simulink model "bench_axle"  (R2024b)
settings: Solver=daessc  StartTime=0.0  StopTime=20  MaxStep=1e-3  RelTol=1e-3
values from neighbouring files (symbols this model uses):
  PN = evalin('base','PN')    [run_bench_string_heat.m]
libraries: fl_lib x11, loco_native_lib x10, nesl_utility x8, sdl_lib x1
settings Model: Creator=BillBeverley  LastModifiedBy=BillBeverley

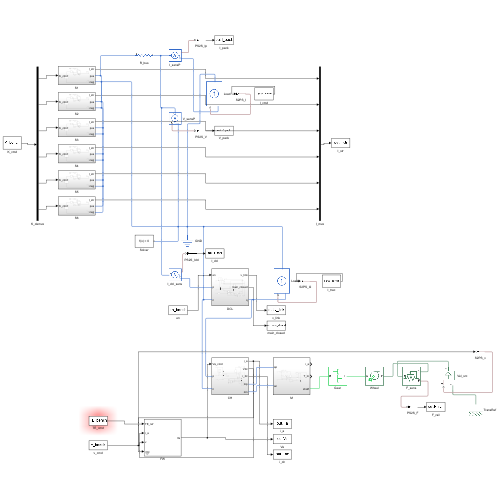
[thumbnail: Simulink's stored preview of the top-level diagram]
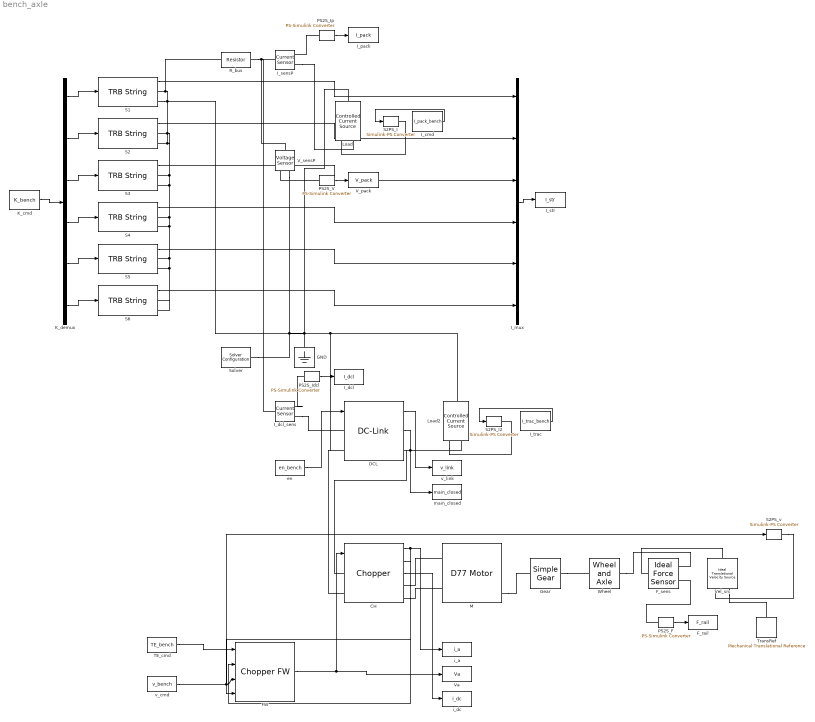
== system bench_axle ==
  CH : loco_native_lib/Chopper  SystemSampleTime=-1  VariantActivationTime=update diagram  AllowFlexibleInterface=on  Latency=0  AutoFrameSizeCalculation=off
  DCL : loco_native_lib/DC-Link  SystemSampleTime=-1  VariantActivationTime=update diagram  AllowFlexibleInterface=on  Latency=0  AutoFrameSizeCalculation=off
  FW : loco_native_lib/Chopper FW  A=PN.ax
  F_rail : ToWorkspace  VariableName=F_rail  SaveFormat=Timeseries  SampleTime=-1
  F_sens : fl_lib/Mechanical/Mechanical Sensors/Ideal Force Sensor
  GND : fl_lib/Electrical/Electrical Elements/Electrical Reference
  Gear : sdl_lib/Gears/Simple Gear  ratio=PN.ax.G  rotation_direction=sdl.enum.shaftOutputDirection.same  friction_model=sdl.enum.gear_efficiencies_load.constant  T_noload=0.1 N*m  T_nom=5 N*m  efficiency_nom=0.8  efficiency=PN.ax.eta_g  temperature_TLU=[280, 300, 320] K  load_TLU=[1, 5, 10] N*m  efficiency_TLU=[.95, .9, .85]  efficiency_TLU2=[.85, .8, .75; .95, .9, .85; .85, .8, .7]  w_thr=0.01 rad/s  pwr_thr=1e3 W  enable_backlash=false  hardstop_model=simscape.enum.hardstop.smooth  backlash_distance=1e-3 mm  r_base=0.1 m  transition=1e-4 mm  backlash_stiffness=1e6 N/m  backlash_damping=1e3 N*s/m  coeff_rest=0.7  v_tol=0.001 m/s  f_tol=0.001 N  mu_visc=[0, 0] N*m*s/rad  thermal_mass=50 J/K  temperature_specify=off  temperature_priority=High  temperature=300 K  temperature_nominal_specify=off  temperature_nominal_value=1  temperature_nominal_unit=K  x_backlash_specify=off  x_backlash_priority=None  x_backlash=0 mm  x_backlash_nominal_specify=off  x_backlash_nominal_value=1  x_backlash_nominal_unit=mm  f_hardstop_specify=off  f_hardstop_priority=None  f_hardstop=0 N  f_hardstop_nominal_specify=off  f_hardstop_nominal_value=1  f_hardstop_nominal_unit=N  v_backlash_specify=off  v_backlash_priority=None  v_backlash=0 m/s  v_backlash_nominal_specify=off  v_backlash_nominal_value=1  v_backlash_nominal_unit=m/s
  I_cmd : FromWorkspace  VariableName=I_pack_bench
  I_dcl : ToWorkspace  VariableName=I_dcl  SaveFormat=Timeseries  SampleTime=-1
  I_dcl_sens : fl_lib/Electrical/Electrical Sensors/Current Sensor
  I_mux : Mux  Inputs=6
  I_pack : ToWorkspace  VariableName=I_pack  SaveFormat=Timeseries  SampleTime=-1
  I_sensP : fl_lib/Electrical/Electrical Sensors/Current Sensor
  I_str : ToWorkspace  VariableName=I_str  SaveFormat=Timeseries  SampleTime=-1
  I_trac : FromWorkspace  VariableName=I_trac_bench
  K_cmd : FromWorkspace  VariableName=K_bench
  K_demux : Demux  Outputs=6
  Load : fl_lib/Electrical/Electrical Sources/Controlled Current Source
  Load2 : fl_lib/Electrical/Electrical Sources/Controlled Current Source
  M : loco_native_lib/D77 Motor  SystemSampleTime=-1  VariantActivationTime=update diagram  AllowFlexibleInterface=on  Latency=0  AutoFrameSizeCalculation=off
  PS2S_F : nesl_utility/PS-Simulink Converter  PhysicalDomain=network_engine_domain  SubClassName=ps_output  LeftPortType=input  RightPortType=output  PseudoPeriodic=off  Frequencies=[]  VectorFormat=inherit  Unit=N  AffineConversion=off
  PS2S_Idcl : nesl_utility/PS-Simulink Converter  PhysicalDomain=network_engine_domain  SubClassName=ps_output  LeftPortType=input  RightPortType=output  PseudoPeriodic=off  Frequencies=[]  VectorFormat=inherit  Unit=A  AffineConversion=off
  PS2S_Ip : nesl_utility/PS-Simulink Converter  PhysicalDomain=network_engine_domain  SubClassName=ps_output  LeftPortType=input  RightPortType=output  PseudoPeriodic=off  Frequencies=[]  VectorFormat=inherit  Unit=A  AffineConversion=off
  PS2S_V : nesl_utility/PS-Simulink Converter  PhysicalDomain=network_engine_domain  SubClassName=ps_output  LeftPortType=input  RightPortType=output  PseudoPeriodic=off  Frequencies=[]  VectorFormat=inherit  Unit=V  AffineConversion=off
  R_bus : fl_lib/Electrical/Electrical Elements/Resistor  R=PN.bus.R Ohm  i_specify=off  i_priority=None  i=0 A  i_nominal_specify=off  i_nominal_value=1  i_nominal_unit=A  v_specify=off  v_priority=None  v=0 V  v_nominal_specify=off  v_nominal_value=1  v_nominal_unit=V
  S{1..6} (6 alike) : loco_native_lib/TRB String  SystemSampleTime=-1  VariantActivationTime=update diagram  AllowFlexibleInterface=on  Latency=0  AutoFrameSizeCalculation=off
  S2PS_I : nesl_utility/Simulink-PS Converter  PhysicalDomain=network_engine_domain  SubClassName=ps_input  LeftPortType=input  RightPortType=output  PseudoPeriodic=off  Frequencies=[]  NoiseDistribution=none  NoiseParameters=[]  Unit=A  AffineConversion=off  FilteringAndDerivatives=provide  SimscapeFilterOrder=1  InputFilterTimeConstant=0.001  UdotUserProvided=0
  S2PS_I2 : nesl_utility/Simulink-PS Converter  PhysicalDomain=network_engine_domain  SubClassName=ps_input  LeftPortType=input  RightPortType=output  PseudoPeriodic=off  Frequencies=[]  NoiseDistribution=none  NoiseParameters=[]  Unit=A  AffineConversion=off  FilteringAndDerivatives=provide  SimscapeFilterOrder=1  InputFilterTimeConstant=0.001  UdotUserProvided=0
  S2PS_v : nesl_utility/Simulink-PS Converter  PhysicalDomain=network_engine_domain  SubClassName=ps_input  LeftPortType=input  RightPortType=output  PseudoPeriodic=off  Frequencies=[]  NoiseDistribution=none  NoiseParameters=[]  Unit=m/s  AffineConversion=off  FilteringAndDerivatives=filter  SimscapeFilterOrder=1  InputFilterTimeConstant=0.001  UdotUserProvided=0
  Solver : nesl_utility/Solver Configuration  PhysicalDomain=network_engine_domain  SubClassName=solver  LeftPortType=input  RightPortType=generic  Tones=[]  Harmonics=[]  SimulateNoise=off  Profile=off  UseLocalSampling=off  EnableSwitchedLinearOptims=on  FrequencyDomain=off  UseCCode=off  RelTol=0.001  AbsTol=0.001  MinStep=1e-09  ToWorkspace=off  RevertToSquareIcSolve=off  NumHomotopyIterations=100  PhasorMode=off  PhasorModeNumHarmonics=1  ConsistencySolver=NEWTON_XTOL_AFTER_FTOL  IndexReductionMethod=DerivativeReplacement  DoDC=off  ResidualTolerance=1e-09  ConsistencyTolSource=GLOBAL  ConsistencyAbsTol=0.001  ConsistencyRelTol=0.001  ConsistencyTolFactor=0.001  UseLocalSolver=off  LocalSolverChoice=NE_BACKWARD_EULER_ADVANCER  ResolveIndetEquations=on  FunctionEvalNumThread=1  LocalSolverSampleTime=0.001  DoFixedCost=off  MaxNonlinIter=3  MaxModeIter=2  ComputeImpulses=off  ImpulseIterations=2  LinearAlgebra=auto  LinearAlgebraNumThread=0  EquationFormulation=NE_TIME_EF  DelaysMemoryBudget=1024  AutomaticFiltering=on  FilteringTimeConstant=0.001  PartitionStorageMethod=AS_NEEDED  PartitionMemoryBudget=1024  PartitionMethod=ROBUST  MultibodyUseLocalSolver=off  MultibodyLocalSolverChoice=ODE1  MultibodyLocalSolverSampleTime=0.001
  TE_cmd : FromWorkspace  VariableName=TE_bench
  TransRef : fl_lib/Mechanical/Translational Elements/Mechanical Translational Reference
  V_pack : ToWorkspace  VariableName=V_pack  SaveFormat=Timeseries  SampleTime=-1
  V_sensP : fl_lib/Electrical/Electrical Sensors/Voltage Sensor
  Va : ToWorkspace  VariableName=Va  SaveFormat=Timeseries  SampleTime=-1
  Vel_src : fl_lib/Mechanical/Mechanical Sources/Ideal Translational Velocity Source
  Wheel : fl_lib/Mechanical/Mechanisms/Wheel and Axle  R=PN.ax.r_w m  or=1  t_specify=off  t_priority=None  t=0 N*m  t_nominal_specify=off  t_nominal_value=1  t_nominal_unit=N*m  f_specify=off  f_priority=None  f=0 N  f_nominal_specify=off  f_nominal_value=1  f_nominal_unit=N
  en : FromWorkspace  VariableName=en_bench
  i_a : ToWorkspace  VariableName=i_a  SaveFormat=Timeseries  SampleTime=-1
  i_dc : ToWorkspace  VariableName=i_dc  SaveFormat=Timeseries  SampleTime=-1
  main_closed : ToWorkspace  VariableName=main_closed  SaveFormat=Timeseries  SampleTime=-1
  v_cmd : FromWorkspace  VariableName=v_bench
  v_link : ToWorkspace  VariableName=v_link  SaveFormat=Timeseries  SampleTime=-1
  wires:
  K_cmd/1 -> K_demux/1
  I_mux/1 -> I_str/1
  K_demux/1 -> S1/1
  S1/1 -> I_mux/1
  K_demux/2 -> S2/1
  S2/1 -> I_mux/2
  K_demux/3 -> S3/1
  S3/1 -> I_mux/3
  K_demux/4 -> S4/1
  S4/1 -> I_mux/4
  K_demux/5 -> S5/1
  S5/1 -> I_mux/5
  K_demux/6 -> S6/1
  S6/1 -> I_mux/6
  I_cmd/1 -> S2PS_I/1
  PS2S_Ip/1 -> I_pack/1
  PS2S_V/1 -> V_pack/1
  I_trac/1 -> S2PS_I2/1
  en/1 -> DCL/1
  DCL/1 -> v_link/1
  DCL/2 -> main_closed/1
  PS2S_Idcl/1 -> I_dcl/1
  TE_cmd/1 -> FW/1
  CH/1 -> FW/2, i_a/1
  v_cmd/1 -> FW/3, S2PS_v/1
  CH/2 -> FW/4
  FW/1 -> CH/1, Va/1
  CH/3 -> i_dc/1
  PS2S_F/1 -> F_rail/1
  connections:
  S1/RConn1 -- R_bus/LConn1 -- S2/RConn1 -- S3/RConn1 -- S4/RConn1 -- S5/RConn1 -- S6/RConn1
  R_bus/RConn1 -- I_dcl_sens/LConn1 -- V_sensP/LConn1 -- I_sensP/LConn1
  I_sensP/RConn2 -- Load/RConn2
  S2PS_I/RConn1 -- Load/RConn1
  PS2S_Ip/LConn1 -- I_sensP/RConn1
  PS2S_V/LConn1 -- V_sensP/RConn1
  S1/RConn2 -- Solver/RConn1 -- DCL/LConn2 -- CH/LConn2 -- Load2/LConn1 -- GND/LConn1 -- Load/LConn1 -- V_sensP/RConn2 -- S2/RConn2 -- S3/RConn2 -- S4/RConn2 -- S5/RConn2 -- S6/RConn2
  I_dcl_sens/RConn1 -- PS2S_Idcl/LConn1
  I_dcl_sens/RConn2 -- DCL/LConn1
  DCL/RConn1 -- CH/LConn1 -- Load2/RConn2
  Load2/RConn1 -- S2PS_I2/RConn1
  CH/RConn1 -- M/LConn1
  CH/RConn2 -- M/LConn2
  M/RConn1 -- Gear/LConn1
  Gear/RConn1 -- Wheel/LConn1
  Wheel/RConn1 -- F_sens/RConn1
  F_sens/LConn1 -- Vel_src/LConn1
  Vel_src/RConn2 -- TransRef/LConn1
  PS2S_F/LConn1 -- F_sens/RConn2
  S2PS_v/RConn1 -- Vel_src/RConn1
